simulink model "ARI_25_1_Smith_predictor"  (Simulink 7.8)
settings: Solver=ode45  StartTime=0.0  StopTime=5  RelTol=1e-3
values from neighbouring files (symbols this model uses):
  tau = tol*max(norm(y,'inf'),1.0)    [phase.m]
undefined symbols (not defined in the file or in its folder): A, B, C, D
libraries: simulink x1
settings Model: Creator=Michael Sebek  ModifiedByFormat=Michael Sebek  LastModifiedBy=Michael Sebek
settings OptimizationCC: InitFltsAndDblsToZero=on
settings DebuggingCC: SaveWithParameterizedLinksMsg=none  SignalResolutionControl=TryResolveAllWithWarning  MultiTaskDSMMsg=warning  MultiTaskCondExecSysMsg=none  FcnCallInpInsideContextMsg=Use local settings  StrictBusMsg=None
settings RTWCC: IncludeERTFirstTime=on
settings GRTTargetCC: TargetFcnLib=ansi_tfl_tmw.mat

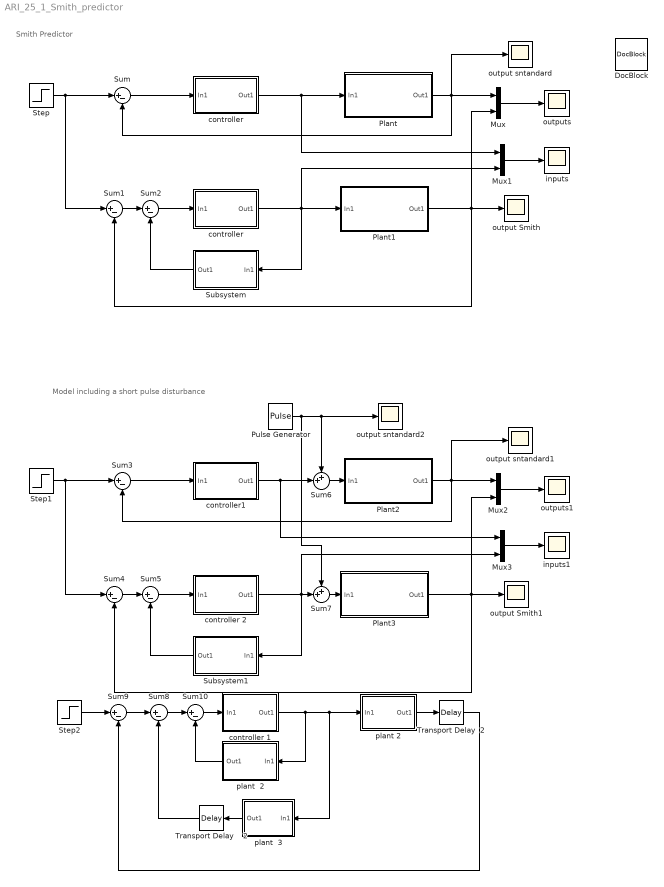
== system ARI_25_1_Smith_predictor ==
  note: Smith Predictor
  note: Model including a short pulse disturbance
  DocBlock : simulink/Model-Wide Utilities/DocBlock  DocumentType=Text
  Mux{,1..3} (4 alike) : Mux  Inputs=2
  Plant : Subsystem
      mask Display: disp('F(s)*exp(-s*tau)')
  Plant1 : Subsystem
      mask Display: disp('F(s)*exp(-s*tau)')
  Plant2 : Subsystem
      mask Display: disp('F(s)*exp(-s*tau)')
  Plant3 : Subsystem
      mask Display: disp('F(s)*exp(-s*tau)')
  Pulse Generator : DiscretePulseGenerator  PulseType=Time based  Period=100  PhaseDelay=1
  Step : Step  Time=0  SampleTime=0
  Step1 : Step  Time=0  SampleTime=0
  Step2 : Step  SampleTime=0
  Subsystem : Subsystem
      mask Display: disp('Smith')
  Subsystem1 : Subsystem
      mask Display: disp('Smith')
  Sum{,1..5,8..10} (9 alike) : Sum  Inputs=|+-
  Sum6 : Sum  Inputs=++|
  Sum7 : Sum  Inputs=++|
  Transport Delay    2 : TransportDelay
  Transport Delay  2 : TransportDelay
  controller : Subsystem  mask(PMF Block){F=C, InCon=[ ], SampTime=1, fvar=No change}
      mask prompts: F "PMF Object:"; InCon "Initial states:"; SampTime "Sample time (discrete time only):"; fvar "Force variable:"
      mask help:
      | Polynomial matrix fraction description of a linear system.
      |
      | This block represents a linear system defined by the polynomial matrix fraction of its transfer function.
      mask init:
      | Label = 'xxx';
      | [A,B,C,D,Label,var] = polymask2(F, fvar, length(InCon));
      | update;
      mask Help:
      | This block represents a linear system [<I>A,B,C,D</I>] defined by the polynomial matrix fraction (<I>PMF</I>) of its transfer function <I>T</I>.
      | <p>
      | <b>Left Matrix Fraction</b> item of the popup menu <b>Type</b> indicates the transfer function in the form of <I>left PMF</I>:
      | <p>
      | <I>T</I> = inv(<I>Q</I>) <I>P</I>.
      | <p>
      | <b>Right Matrix Fraction</b> item is used if the transfer function is given in the form of <I>right PMF</I>:
      | <p>
      | <I>T</I> = <I>P</I> inv(<I>Q</I>).
      | <p>
      |  The <b>variable</b> determines the type  of the system:
      | <p>
      | - <b>s, p</b> are used for continous time systems (Laplace transform).
      | <p>
      | - <b>z, q</b> are used for discrete time transfer functions in forward-shift operator (Z-transform).
      | <p>
      | - <b>d, z^-1</b> are used for discrete time transfer functions in backward-shift operator.
      | <p>
      | <b> Note:</b> For the variables <I>s,p,z,q</I>, the transfer function is defined as
      | <p>
      | <I>T</I> = <I>C</I> inv(<I>vI-A</I>) <I>B</I> + <I>D</I>,
      | <p>
      | where <I>v</I> is the variable of <I>P,Q</I>.
      | For the variables <I>d, z^-1</I>, the transfer function is defined as
      | <p>
      | <I>T</I> = <I>C v</I> inv(<I>I-Av</I>)  <I>B</I> + <I>D</I>.
      | <p>
      | <b>Note:</b> <b>Initial states</b> concern the observer-form realization of the system as defined by LMF2S and RMF2S functions. Their number must equal the sum of column degrees of the denominator matrix <I>Q</I> in case of right PMF and the sum of row degrees of <I>Q</I> for left PMF description.
      | <p>
      | See also POL, LMF2S, RMF2S.
      mask StyleString: edit,edit,edit,popup(No change|s   (continous time)|p   (continous time)|z      (discrete time)|q      (discrete time)|d      (discrete time)|z^-1 (discrete time))
      mask Display: disp('C(s)')
  "controller " : Subsystem  mask(PMF Block){F=C, InCon=[ ], SampTime=1, fvar=No change}
      mask prompts: F "PMF Object:"; InCon "Initial states:"; SampTime "Sample time (discrete time only):"; fvar "Force variable:"
      mask help:
      | Polynomial matrix fraction description of a linear system.
      |
      | This block represents a linear system defined by the polynomial matrix fraction of its transfer function.
      mask init:
      | Label = 'xxx';
      | [A,B,C,D,Label,var] = polymask2(F, fvar, length(InCon));
      | update;
      mask Help:
      | This block represents a linear system [<I>A,B,C,D</I>] defined by the polynomial matrix fraction (<I>PMF</I>) of its transfer function <I>T</I>.
      | <p>
      | <b>Left Matrix Fraction</b> item of the popup menu <b>Type</b> indicates the transfer function in the form of <I>left PMF</I>:
      | <p>
      | <I>T</I> = inv(<I>Q</I>) <I>P</I>.
      | <p>
      | <b>Right Matrix Fraction</b> item is used if the transfer function is given in the form of <I>right PMF</I>:
      | <p>
      | <I>T</I> = <I>P</I> inv(<I>Q</I>).
      | <p>
      |  The <b>variable</b> determines the type  of the system:
      | <p>
      | - <b>s, p</b> are used for continous time systems (Laplace transform).
      | <p>
      | - <b>z, q</b> are used for discrete time transfer functions in forward-shift operator (Z-transform).
      | <p>
      | - <b>d, z^-1</b> are used for discrete time transfer functions in backward-shift operator.
      | <p>
      | <b> Note:</b> For the variables <I>s,p,z,q</I>, the transfer function is defined as
      | <p>
      | <I>T</I> = <I>C</I> inv(<I>vI-A</I>) <I>B</I> + <I>D</I>,
      | <p>
      | where <I>v</I> is the variable of <I>P,Q</I>.
      | For the variables <I>d, z^-1</I>, the transfer function is defined as
      | <p>
      | <I>T</I> = <I>C v</I> inv(<I>I-Av</I>)  <I>B</I> + <I>D</I>.
      | <p>
      | <b>Note:</b> <b>Initial states</b> concern the observer-form realization of the system as defined by LMF2S and RMF2S functions. Their number must equal the sum of column degrees of the denominator matrix <I>Q</I> in case of right PMF and the sum of row degrees of <I>Q</I> for left PMF description.
      | <p>
      | See also POL, LMF2S, RMF2S.
      mask StyleString: edit,edit,edit,popup(No change|s   (continous time)|p   (continous time)|z      (discrete time)|q      (discrete time)|d      (discrete time)|z^-1 (discrete time))
      mask Display: disp('C(s)')
  controller 1 : Subsystem  mask(PMF Block){F=1/s, InCon=[ ], SampTime=1, fvar=No change}
      mask prompts: F "PMF Object:"; InCon "Initial states:"; SampTime "Sample time (discrete time only):"; fvar "Force variable:"
      mask help:
      | Polynomial matrix fraction description of a linear system.
      |
      | This block represents a linear system defined by the polynomial matrix fraction of its transfer function.
      mask init:
      | Label = 'xxx';
      | [A,B,C,D,Label,var] = polymask2(F, fvar, length(InCon));
      | update;
      mask Help:
      | This block represents a linear system [<I>A,B,C,D</I>] defined by the polynomial matrix fraction (<I>PMF</I>) of its transfer function <I>T</I>.
      | <p>
      | <b>Left Matrix Fraction</b> item of the popup menu <b>Type</b> indicates the transfer function in the form of <I>left PMF</I>:
      | <p>
      | <I>T</I> = inv(<I>Q</I>) <I>P</I>.
      | <p>
      | <b>Right Matrix Fraction</b> item is used if the transfer function is given in the form of <I>right PMF</I>:
      | <p>
      | <I>T</I> = <I>P</I> inv(<I>Q</I>).
      | <p>
      |  The <b>variable</b> determines the type  of the system:
      | <p>
      | - <b>s, p</b> are used for continous time systems (Laplace transform).
      | <p>
      | - <b>z, q</b> are used for discrete time transfer functions in forward-shift operator (Z-transform).
      | <p>
      | - <b>d, z^-1</b> are used for discrete time transfer functions in backward-shift operator.
      | <p>
      | <b> Note:</b> For the variables <I>s,p,z,q</I>, the transfer function is defined as
      | <p>
      | <I>T</I> = <I>C</I> inv(<I>vI-A</I>) <I>B</I> + <I>D</I>,
      | <p>
      | where <I>v</I> is the variable of <I>P,Q</I>.
      | For the variables <I>d, z^-1</I>, the transfer function is defined as
      | <p>
      | <I>T</I> = <I>C v</I> inv(<I>I-Av</I>)  <I>B</I> + <I>D</I>.
      | <p>
      | <b>Note:</b> <b>Initial states</b> concern the observer-form realization of the system as defined by LMF2S and RMF2S functions. Their number must equal the sum of column degrees of the denominator matrix <I>Q</I> in case of right PMF and the sum of row degrees of <I>Q</I> for left PMF description.
      | <p>
      | See also POL, LMF2S, RMF2S.
      mask StyleString: edit,edit,edit,popup(No change|s   (continous time)|p   (continous time)|z      (discrete time)|q      (discrete time)|d      (discrete time)|z^-1 (discrete time))
      mask Display: disp(Label);
  controller 2 : Subsystem  mask(PMF Block){F=C, InCon=[ ], SampTime=1, fvar=No change}
      mask prompts: F "PMF Object:"; InCon "Initial states:"; SampTime "Sample time (discrete time only):"; fvar "Force variable:"
      mask help:
      | Polynomial matrix fraction description of a linear system.
      |
      | This block represents a linear system defined by the polynomial matrix fraction of its transfer function.
      mask init:
      | Label = 'xxx';
      | [A,B,C,D,Label,var] = polymask2(F, fvar, length(InCon));
      | update;
      mask Help:
      | This block represents a linear system [<I>A,B,C,D</I>] defined by the polynomial matrix fraction (<I>PMF</I>) of its transfer function <I>T</I>.
      | <p>
      | <b>Left Matrix Fraction</b> item of the popup menu <b>Type</b> indicates the transfer function in the form of <I>left PMF</I>:
      | <p>
      | <I>T</I> = inv(<I>Q</I>) <I>P</I>.
      | <p>
      | <b>Right Matrix Fraction</b> item is used if the transfer function is given in the form of <I>right PMF</I>:
      | <p>
      | <I>T</I> = <I>P</I> inv(<I>Q</I>).
      | <p>
      |  The <b>variable</b> determines the type  of the system:
      | <p>
      | - <b>s, p</b> are used for continous time systems (Laplace transform).
      | <p>
      | - <b>z, q</b> are used for discrete time transfer functions in forward-shift operator (Z-transform).
      | <p>
      | - <b>d, z^-1</b> are used for discrete time transfer functions in backward-shift operator.
      | <p>
      | <b> Note:</b> For the variables <I>s,p,z,q</I>, the transfer function is defined as
      | <p>
      | <I>T</I> = <I>C</I> inv(<I>vI-A</I>) <I>B</I> + <I>D</I>,
      | <p>
      | where <I>v</I> is the variable of <I>P,Q</I>.
      | For the variables <I>d, z^-1</I>, the transfer function is defined as
      | <p>
      | <I>T</I> = <I>C v</I> inv(<I>I-Av</I>)  <I>B</I> + <I>D</I>.
      | <p>
      | <b>Note:</b> <b>Initial states</b> concern the observer-form realization of the system as defined by LMF2S and RMF2S functions. Their number must equal the sum of column degrees of the denominator matrix <I>Q</I> in case of right PMF and the sum of row degrees of <I>Q</I> for left PMF description.
      | <p>
      | See also POL, LMF2S, RMF2S.
      mask StyleString: edit,edit,edit,popup(No change|s   (continous time)|p   (continous time)|z      (discrete time)|q      (discrete time)|d      (discrete time)|z^-1 (discrete time))
      mask Display: disp('C(s)')
  controller1 : Subsystem  mask(PMF Block){F=C, InCon=[ ], SampTime=1, fvar=No change}
      mask prompts: F "PMF Object:"; InCon "Initial states:"; SampTime "Sample time (discrete time only):"; fvar "Force variable:"
      mask help:
      | Polynomial matrix fraction description of a linear system.
      |
      | This block represents a linear system defined by the polynomial matrix fraction of its transfer function.
      mask init:
      | Label = 'xxx';
      | [A,B,C,D,Label,var] = polymask2(F, fvar, length(InCon));
      | update;
      mask Help:
      | This block represents a linear system [<I>A,B,C,D</I>] defined by the polynomial matrix fraction (<I>PMF</I>) of its transfer function <I>T</I>.
      | <p>
      | <b>Left Matrix Fraction</b> item of the popup menu <b>Type</b> indicates the transfer function in the form of <I>left PMF</I>:
      | <p>
      | <I>T</I> = inv(<I>Q</I>) <I>P</I>.
      | <p>
      | <b>Right Matrix Fraction</b> item is used if the transfer function is given in the form of <I>right PMF</I>:
      | <p>
      | <I>T</I> = <I>P</I> inv(<I>Q</I>).
      | <p>
      |  The <b>variable</b> determines the type  of the system:
      | <p>
      | - <b>s, p</b> are used for continous time systems (Laplace transform).
      | <p>
      | - <b>z, q</b> are used for discrete time transfer functions in forward-shift operator (Z-transform).
      | <p>
      | - <b>d, z^-1</b> are used for discrete time transfer functions in backward-shift operator.
      | <p>
      | <b> Note:</b> For the variables <I>s,p,z,q</I>, the transfer function is defined as
      | <p>
      | <I>T</I> = <I>C</I> inv(<I>vI-A</I>) <I>B</I> + <I>D</I>,
      | <p>
      | where <I>v</I> is the variable of <I>P,Q</I>.
      | For the variables <I>d, z^-1</I>, the transfer function is defined as
      | <p>
      | <I>T</I> = <I>C v</I> inv(<I>I-Av</I>)  <I>B</I> + <I>D</I>.
      | <p>
      | <b>Note:</b> <b>Initial states</b> concern the observer-form realization of the system as defined by LMF2S and RMF2S functions. Their number must equal the sum of column degrees of the denominator matrix <I>Q</I> in case of right PMF and the sum of row degrees of <I>Q</I> for left PMF description.
      | <p>
      | See also POL, LMF2S, RMF2S.
      mask StyleString: edit,edit,edit,popup(No change|s   (continous time)|p   (continous time)|z      (discrete time)|q      (discrete time)|d      (discrete time)|z^-1 (discrete time))
      mask Display: disp('C(s)')
  inputs : Scope
      settings: SaveName=ScopeData2
  inputs1 : Scope
      settings: SaveName=ScopeData4
  output Smith : Scope
  output Smith1 : Scope
      settings: SaveName=ScopeData5
  output sntandard : Scope
      settings: SaveName=ScopeData3
  output sntandard1 : Scope
      settings: SaveName=ScopeData6
  output sntandard2 : Scope
      settings: SaveName=ScopeData8
  outputs : Scope
      settings: TimeRange=50  YMin=0  YMax=1.4e+021
  outputs1 : Scope
      settings: TimeRange=50  YMin=0  YMax=1.4e+021  SaveName=ScopeData7
  plant  2 : Subsystem  mask(PMF Block){F=rdf(1,s+1), InCon=[ ], SampTime=1, fvar=No change}
      mask prompts: F "PMF Object:"; InCon "Initial states:"; SampTime "Sample time (discrete time only):"; fvar "Force variable:"
      mask help:
      | Polynomial matrix fraction description of a linear system.
      |
      | This block represents a linear system defined by the polynomial matrix fraction of its transfer function.
      mask init:
      | Label = 'xxx';
      | [A,B,C,D,Label,var] = polymask2(F, fvar, length(InCon));
      | update;
      mask Help:
      | This block represents a linear system [<I>A,B,C,D</I>] defined by the polynomial matrix fraction (<I>PMF</I>) of its transfer function <I>T</I>.
      | <p>
      | <b>Left Matrix Fraction</b> item of the popup menu <b>Type</b> indicates the transfer function in the form of <I>left PMF</I>:
      | <p>
      | <I>T</I> = inv(<I>Q</I>) <I>P</I>.
      | <p>
      | <b>Right Matrix Fraction</b> item is used if the transfer function is given in the form of <I>right PMF</I>:
      | <p>
      | <I>T</I> = <I>P</I> inv(<I>Q</I>).
      | <p>
      |  The <b>variable</b> determines the type  of the system:
      | <p>
      | - <b>s, p</b> are used for continous time systems (Laplace transform).
      | <p>
      | - <b>z, q</b> are used for discrete time transfer functions in forward-shift operator (Z-transform).
      | <p>
      | - <b>d, z^-1</b> are used for discrete time transfer functions in backward-shift operator.
      | <p>
      | <b> Note:</b> For the variables <I>s,p,z,q</I>, the transfer function is defined as
      | <p>
      | <I>T</I> = <I>C</I> inv(<I>vI-A</I>) <I>B</I> + <I>D</I>,
      | <p>
      | where <I>v</I> is the variable of <I>P,Q</I>.
      | For the variables <I>d, z^-1</I>, the transfer function is defined as
      | <p>
      | <I>T</I> = <I>C v</I> inv(<I>I-Av</I>)  <I>B</I> + <I>D</I>.
      | <p>
      | <b>Note:</b> <b>Initial states</b> concern the observer-form realization of the system as defined by LMF2S and RMF2S functions. Their number must equal the sum of column degrees of the denominator matrix <I>Q</I> in case of right PMF and the sum of row degrees of <I>Q</I> for left PMF description.
      | <p>
      | See also POL, LMF2S, RMF2S.
      mask StyleString: edit,edit,edit,popup(No change|s   (continous time)|p   (continous time)|z      (discrete time)|q      (discrete time)|d      (discrete time)|z^-1 (discrete time))
      mask Display: disp(Label);
  plant  3 : Subsystem  mask(PMF Block){F=rdf(1,s+1), InCon=[ ], SampTime=1, fvar=No change}
      mask prompts: F "PMF Object:"; InCon "Initial states:"; SampTime "Sample time (discrete time only):"; fvar "Force variable:"
      mask help:
      | Polynomial matrix fraction description of a linear system.
      |
      | This block represents a linear system defined by the polynomial matrix fraction of its transfer function.
      mask init:
      | Label = 'xxx';
      | [A,B,C,D,Label,var] = polymask2(F, fvar, length(InCon));
      | update;
      mask Help:
      | This block represents a linear system [<I>A,B,C,D</I>] defined by the polynomial matrix fraction (<I>PMF</I>) of its transfer function <I>T</I>.
      | <p>
      | <b>Left Matrix Fraction</b> item of the popup menu <b>Type</b> indicates the transfer function in the form of <I>left PMF</I>:
      | <p>
      | <I>T</I> = inv(<I>Q</I>) <I>P</I>.
      | <p>
      | <b>Right Matrix Fraction</b> item is used if the transfer function is given in the form of <I>right PMF</I>:
      | <p>
      | <I>T</I> = <I>P</I> inv(<I>Q</I>).
      | <p>
      |  The <b>variable</b> determines the type  of the system:
      | <p>
      | - <b>s, p</b> are used for continous time systems (Laplace transform).
      | <p>
      | - <b>z, q</b> are used for discrete time transfer functions in forward-shift operator (Z-transform).
      | <p>
      | - <b>d, z^-1</b> are used for discrete time transfer functions in backward-shift operator.
      | <p>
      | <b> Note:</b> For the variables <I>s,p,z,q</I>, the transfer function is defined as
      | <p>
      | <I>T</I> = <I>C</I> inv(<I>vI-A</I>) <I>B</I> + <I>D</I>,
      | <p>
      | where <I>v</I> is the variable of <I>P,Q</I>.
      | For the variables <I>d, z^-1</I>, the transfer function is defined as
      | <p>
      | <I>T</I> = <I>C v</I> inv(<I>I-Av</I>)  <I>B</I> + <I>D</I>.
      | <p>
      | <b>Note:</b> <b>Initial states</b> concern the observer-form realization of the system as defined by LMF2S and RMF2S functions. Their number must equal the sum of column degrees of the denominator matrix <I>Q</I> in case of right PMF and the sum of row degrees of <I>Q</I> for left PMF description.
      | <p>
      | See also POL, LMF2S, RMF2S.
      mask StyleString: edit,edit,edit,popup(No change|s   (continous time)|p   (continous time)|z      (discrete time)|q      (discrete time)|d      (discrete time)|z^-1 (discrete time))
      mask Display: disp(Label);
  plant 2 : Subsystem  mask(PMF Block){F=rdf(1,s+1), InCon=[ ], SampTime=1, fvar=No change}
      mask prompts: F "PMF Object:"; InCon "Initial states:"; SampTime "Sample time (discrete time only):"; fvar "Force variable:"
      mask help:
      | Polynomial matrix fraction description of a linear system.
      |
      | This block represents a linear system defined by the polynomial matrix fraction of its transfer function.
      mask init:
      | Label = 'xxx';
      | [A,B,C,D,Label,var] = polymask2(F, fvar, length(InCon));
      | update;
      mask Help:
      | This block represents a linear system [<I>A,B,C,D</I>] defined by the polynomial matrix fraction (<I>PMF</I>) of its transfer function <I>T</I>.
      | <p>
      | <b>Left Matrix Fraction</b> item of the popup menu <b>Type</b> indicates the transfer function in the form of <I>left PMF</I>:
      | <p>
      | <I>T</I> = inv(<I>Q</I>) <I>P</I>.
      | <p>
      | <b>Right Matrix Fraction</b> item is used if the transfer function is given in the form of <I>right PMF</I>:
      | <p>
      | <I>T</I> = <I>P</I> inv(<I>Q</I>).
      | <p>
      |  The <b>variable</b> determines the type  of the system:
      | <p>
      | - <b>s, p</b> are used for continous time systems (Laplace transform).
      | <p>
      | - <b>z, q</b> are used for discrete time transfer functions in forward-shift operator (Z-transform).
      | <p>
      | - <b>d, z^-1</b> are used for discrete time transfer functions in backward-shift operator.
      | <p>
      | <b> Note:</b> For the variables <I>s,p,z,q</I>, the transfer function is defined as
      | <p>
      | <I>T</I> = <I>C</I> inv(<I>vI-A</I>) <I>B</I> + <I>D</I>,
      | <p>
      | where <I>v</I> is the variable of <I>P,Q</I>.
      | For the variables <I>d, z^-1</I>, the transfer function is defined as
      | <p>
      | <I>T</I> = <I>C v</I> inv(<I>I-Av</I>)  <I>B</I> + <I>D</I>.
      | <p>
      | <b>Note:</b> <b>Initial states</b> concern the observer-form realization of the system as defined by LMF2S and RMF2S functions. Their number must equal the sum of column degrees of the denominator matrix <I>Q</I> in case of right PMF and the sum of row degrees of <I>Q</I> for left PMF description.
      | <p>
      | See also POL, LMF2S, RMF2S.
      mask StyleString: edit,edit,edit,popup(No change|s   (continous time)|p   (continous time)|z      (discrete time)|q      (discrete time)|d      (discrete time)|z^-1 (discrete time))
      mask Display: droots([], [-1], 1)
  wires:
  Mux/1 -> outputs/1
  Plant/1(Out1) -> Mux/1, Sum/2, output sntandard/1
  controller/1(Out1) -> Plant/1(In1), Mux1/1
  Sum/1 -> controller/1(In1)
  Step/1 -> Sum/1, Sum1/1
  "controller "/1(Out1) -> Plant1/1(In1), Subsystem/1(In1), Mux1/2
  Sum2/1 -> "controller "/1(In1)
  Subsystem/1(Out1) -> Sum2/2
  plant 2/1(Out1) -> Transport Delay  2/1
  controller 1/1(Out1) -> plant  2/1(In1), plant 2/1(In1), plant  3/1(In1)
  Sum10/1 -> controller 1/1(In1)
  plant  2/1(Out1) -> Sum10/2
  Transport Delay  2/1 -> Sum9/2
  Step2/1 -> Sum9/1
  plant  3/1(Out1) -> Transport Delay    2/1
  Sum8/1 -> Sum10/1
  Sum9/1 -> Sum8/1
  Transport Delay    2/1 -> Sum8/2
  Plant1/1(Out1) -> Sum1/2, output Smith/1, Mux/2
  Mux1/1 -> inputs/1
  Sum1/1 -> Sum2/1
  Mux2/1 -> outputs1/1
  Plant2/1(Out1) -> output sntandard1/1, Sum3/2, Mux2/1
  Sum3/1 -> controller1/1(In1)
  Step1/1 -> Sum4/1, Sum3/1
  Sum5/1 -> controller 2/1(In1)
  Subsystem1/1(Out1) -> Sum5/2
  Plant3/1(Out1) -> Mux2/2, output Smith1/1, Sum4/2
  Mux3/1 -> inputs1/1
  Sum4/1 -> Sum5/1
  controller1/1(Out1) -> Sum6/2, Mux3/1
  Sum6/1 -> Plant2/1(In1)
  Pulse Generator/1 -> Sum6/1, output sntandard2/1, Sum7/1
  controller 2/1(Out1) -> Mux3/2, Subsystem1/1(In1), Sum7/2
  Sum7/1 -> Plant3/1(In1)

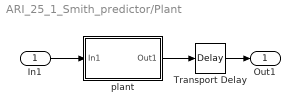
== system ARI_25_1_Smith_predictor/Plant ==
  In1 : Inport
  Transport Delay : TransportDelay  DelayTime=tau
  plant : Subsystem  mask(PMF Block){F=F, InCon=[ ], SampTime=1, fvar=No change}
      mask prompts: F "PMF Object:"; InCon "Initial states:"; SampTime "Sample time (discrete time only):"; fvar "Force variable:"
      mask help:
      | Polynomial matrix fraction description of a linear system.
      |
      | This block represents a linear system defined by the polynomial matrix fraction of its transfer function.
      mask init:
      | Label = 'xxx';
      | [A,B,C,D,Label,var] = polymask2(F, fvar, length(InCon));
      | update;
      mask Help:
      | This block represents a linear system [<I>A,B,C,D</I>] defined by the polynomial matrix fraction (<I>PMF</I>) of its transfer function <I>T</I>.
      | <p>
      | <b>Left Matrix Fraction</b> item of the popup menu <b>Type</b> indicates the transfer function in the form of <I>left PMF</I>:
      | <p>
      | <I>T</I> = inv(<I>Q</I>) <I>P</I>.
      | <p>
      | <b>Right Matrix Fraction</b> item is used if the transfer function is given in the form of <I>right PMF</I>:
      | <p>
      | <I>T</I> = <I>P</I> inv(<I>Q</I>).
      | <p>
      |  The <b>variable</b> determines the type  of the system:
      | <p>
      | - <b>s, p</b> are used for continous time systems (Laplace transform).
      | <p>
      | - <b>z, q</b> are used for discrete time transfer functions in forward-shift operator (Z-transform).
      | <p>
      | - <b>d, z^-1</b> are used for discrete time transfer functions in backward-shift operator.
      | <p>
      | <b> Note:</b> For the variables <I>s,p,z,q</I>, the transfer function is defined as
      | <p>
      | <I>T</I> = <I>C</I> inv(<I>vI-A</I>) <I>B</I> + <I>D</I>,
      | <p>
      | where <I>v</I> is the variable of <I>P,Q</I>.
      | For the variables <I>d, z^-1</I>, the transfer function is defined as
      | <p>
      | <I>T</I> = <I>C v</I> inv(<I>I-Av</I>)  <I>B</I> + <I>D</I>.
      | <p>
      | <b>Note:</b> <b>Initial states</b> concern the observer-form realization of the system as defined by LMF2S and RMF2S functions. Their number must equal the sum of column degrees of the denominator matrix <I>Q</I> in case of right PMF and the sum of row degrees of <I>Q</I> for left PMF description.
      | <p>
      | See also POL, LMF2S, RMF2S.
      mask StyleString: edit,edit,edit,popup(No change|s   (continous time)|p   (continous time)|z      (discrete time)|q      (discrete time)|d      (discrete time)|z^-1 (discrete time))
      mask Display: disp('F(s)')
  Out1 : Outport
  wires:
  plant/1(Out1) -> Transport Delay/1
  In1/1 -> plant/1(In1)
  Transport Delay/1 -> Out1/1

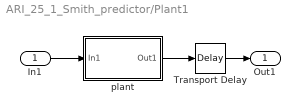
== system ARI_25_1_Smith_predictor/Plant1 ==
  In1 : Inport
  Transport Delay : TransportDelay  DelayTime=tau
  plant : Subsystem  mask(PMF Block){F=F, InCon=[ ], SampTime=1, fvar=No change}
      mask prompts: F "PMF Object:"; InCon "Initial states:"; SampTime "Sample time (discrete time only):"; fvar "Force variable:"
      mask help:
      | Polynomial matrix fraction description of a linear system.
      |
      | This block represents a linear system defined by the polynomial matrix fraction of its transfer function.
      mask init:
      | Label = 'xxx';
      | [A,B,C,D,Label,var] = polymask2(F, fvar, length(InCon));
      | update;
      mask Help:
      | This block represents a linear system [<I>A,B,C,D</I>] defined by the polynomial matrix fraction (<I>PMF</I>) of its transfer function <I>T</I>.
      | <p>
      | <b>Left Matrix Fraction</b> item of the popup menu <b>Type</b> indicates the transfer function in the form of <I>left PMF</I>:
      | <p>
      | <I>T</I> = inv(<I>Q</I>) <I>P</I>.
      | <p>
      | <b>Right Matrix Fraction</b> item is used if the transfer function is given in the form of <I>right PMF</I>:
      | <p>
      | <I>T</I> = <I>P</I> inv(<I>Q</I>).
      | <p>
      |  The <b>variable</b> determines the type  of the system:
      | <p>
      | - <b>s, p</b> are used for continous time systems (Laplace transform).
      | <p>
      | - <b>z, q</b> are used for discrete time transfer functions in forward-shift operator (Z-transform).
      | <p>
      | - <b>d, z^-1</b> are used for discrete time transfer functions in backward-shift operator.
      | <p>
      | <b> Note:</b> For the variables <I>s,p,z,q</I>, the transfer function is defined as
      | <p>
      | <I>T</I> = <I>C</I> inv(<I>vI-A</I>) <I>B</I> + <I>D</I>,
      | <p>
      | where <I>v</I> is the variable of <I>P,Q</I>.
      | For the variables <I>d, z^-1</I>, the transfer function is defined as
      | <p>
      | <I>T</I> = <I>C v</I> inv(<I>I-Av</I>)  <I>B</I> + <I>D</I>.
      | <p>
      | <b>Note:</b> <b>Initial states</b> concern the observer-form realization of the system as defined by LMF2S and RMF2S functions. Their number must equal the sum of column degrees of the denominator matrix <I>Q</I> in case of right PMF and the sum of row degrees of <I>Q</I> for left PMF description.
      | <p>
      | See also POL, LMF2S, RMF2S.
      mask StyleString: edit,edit,edit,popup(No change|s   (continous time)|p   (continous time)|z      (discrete time)|q      (discrete time)|d      (discrete time)|z^-1 (discrete time))
      mask Display: disp('b/a')
  Out1 : Outport
  wires:
  Transport Delay/1 -> Out1/1
  In1/1 -> plant/1(In1)
  plant/1(Out1) -> Transport Delay/1

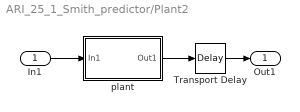
== system ARI_25_1_Smith_predictor/Plant2 ==
  In1 : Inport
  Transport Delay : TransportDelay  DelayTime=tau
  plant : Subsystem  mask(PMF Block){F=F, InCon=[ ], SampTime=1, fvar=No change}
      mask prompts: F "PMF Object:"; InCon "Initial states:"; SampTime "Sample time (discrete time only):"; fvar "Force variable:"
      mask help:
      | Polynomial matrix fraction description of a linear system.
      |
      | This block represents a linear system defined by the polynomial matrix fraction of its transfer function.
      mask init:
      | Label = 'xxx';
      | [A,B,C,D,Label,var] = polymask2(F, fvar, length(InCon));
      | update;
      mask Help:
      | This block represents a linear system [<I>A,B,C,D</I>] defined by the polynomial matrix fraction (<I>PMF</I>) of its transfer function <I>T</I>.
      | <p>
      | <b>Left Matrix Fraction</b> item of the popup menu <b>Type</b> indicates the transfer function in the form of <I>left PMF</I>:
      | <p>
      | <I>T</I> = inv(<I>Q</I>) <I>P</I>.
      | <p>
      | <b>Right Matrix Fraction</b> item is used if the transfer function is given in the form of <I>right PMF</I>:
      | <p>
      | <I>T</I> = <I>P</I> inv(<I>Q</I>).
      | <p>
      |  The <b>variable</b> determines the type  of the system:
      | <p>
      | - <b>s, p</b> are used for continous time systems (Laplace transform).
      | <p>
      | - <b>z, q</b> are used for discrete time transfer functions in forward-shift operator (Z-transform).
      | <p>
      | - <b>d, z^-1</b> are used for discrete time transfer functions in backward-shift operator.
      | <p>
      | <b> Note:</b> For the variables <I>s,p,z,q</I>, the transfer function is defined as
      | <p>
      | <I>T</I> = <I>C</I> inv(<I>vI-A</I>) <I>B</I> + <I>D</I>,
      | <p>
      | where <I>v</I> is the variable of <I>P,Q</I>.
      | For the variables <I>d, z^-1</I>, the transfer function is defined as
      | <p>
      | <I>T</I> = <I>C v</I> inv(<I>I-Av</I>)  <I>B</I> + <I>D</I>.
      | <p>
      | <b>Note:</b> <b>Initial states</b> concern the observer-form realization of the system as defined by LMF2S and RMF2S functions. Their number must equal the sum of column degrees of the denominator matrix <I>Q</I> in case of right PMF and the sum of row degrees of <I>Q</I> for left PMF description.
      | <p>
      | See also POL, LMF2S, RMF2S.
      mask StyleString: edit,edit,edit,popup(No change|s   (continous time)|p   (continous time)|z      (discrete time)|q      (discrete time)|d      (discrete time)|z^-1 (discrete time))
      mask Display: disp('F(s)')
  Out1 : Outport
  wires:
  Transport Delay/1 -> Out1/1
  In1/1 -> plant/1(In1)
  plant/1(Out1) -> Transport Delay/1

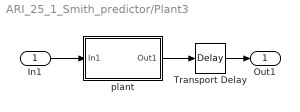
== system ARI_25_1_Smith_predictor/Plant3 ==
  In1 : Inport
  Transport Delay : TransportDelay  DelayTime=tau
  plant : Subsystem  mask(PMF Block){F=F, InCon=[ ], SampTime=1, fvar=No change}
      mask prompts: F "PMF Object:"; InCon "Initial states:"; SampTime "Sample time (discrete time only):"; fvar "Force variable:"
      mask help:
      | Polynomial matrix fraction description of a linear system.
      |
      | This block represents a linear system defined by the polynomial matrix fraction of its transfer function.
      mask init:
      | Label = 'xxx';
      | [A,B,C,D,Label,var] = polymask2(F, fvar, length(InCon));
      | update;
      mask Help:
      | This block represents a linear system [<I>A,B,C,D</I>] defined by the polynomial matrix fraction (<I>PMF</I>) of its transfer function <I>T</I>.
      | <p>
      | <b>Left Matrix Fraction</b> item of the popup menu <b>Type</b> indicates the transfer function in the form of <I>left PMF</I>:
      | <p>
      | <I>T</I> = inv(<I>Q</I>) <I>P</I>.
      | <p>
      | <b>Right Matrix Fraction</b> item is used if the transfer function is given in the form of <I>right PMF</I>:
      | <p>
      | <I>T</I> = <I>P</I> inv(<I>Q</I>).
      | <p>
      |  The <b>variable</b> determines the type  of the system:
      | <p>
      | - <b>s, p</b> are used for continous time systems (Laplace transform).
      | <p>
      | - <b>z, q</b> are used for discrete time transfer functions in forward-shift operator (Z-transform).
      | <p>
      | - <b>d, z^-1</b> are used for discrete time transfer functions in backward-shift operator.
      | <p>
      | <b> Note:</b> For the variables <I>s,p,z,q</I>, the transfer function is defined as
      | <p>
      | <I>T</I> = <I>C</I> inv(<I>vI-A</I>) <I>B</I> + <I>D</I>,
      | <p>
      | where <I>v</I> is the variable of <I>P,Q</I>.
      | For the variables <I>d, z^-1</I>, the transfer function is defined as
      | <p>
      | <I>T</I> = <I>C v</I> inv(<I>I-Av</I>)  <I>B</I> + <I>D</I>.
      | <p>
      | <b>Note:</b> <b>Initial states</b> concern the observer-form realization of the system as defined by LMF2S and RMF2S functions. Their number must equal the sum of column degrees of the denominator matrix <I>Q</I> in case of right PMF and the sum of row degrees of <I>Q</I> for left PMF description.
      | <p>
      | See also POL, LMF2S, RMF2S.
      mask StyleString: edit,edit,edit,popup(No change|s   (continous time)|p   (continous time)|z      (discrete time)|q      (discrete time)|d      (discrete time)|z^-1 (discrete time))
      mask Display: disp('b/a')
  Out1 : Outport
  wires:
  plant/1(Out1) -> Transport Delay/1
  In1/1 -> plant/1(In1)
  Transport Delay/1 -> Out1/1

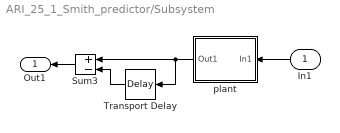
== system ARI_25_1_Smith_predictor/Subsystem ==
  In1 : Inport
  Sum3 : Sum  Inputs=+-
  "Transport Delay    " : TransportDelay  DelayTime=tau
  "plant  " : Subsystem  mask(PMF Block){F=F, InCon=[ ], SampTime=1, fvar=No change}
      mask prompts: F "PMF Object:"; InCon "Initial states:"; SampTime "Sample time (discrete time only):"; fvar "Force variable:"
      mask help:
      | Polynomial matrix fraction description of a linear system.
      |
      | This block represents a linear system defined by the polynomial matrix fraction of its transfer function.
      mask init:
      | Label = 'xxx';
      | [A,B,C,D,Label,var] = polymask2(F, fvar, length(InCon));
      | update;
      mask Help:
      | This block represents a linear system [<I>A,B,C,D</I>] defined by the polynomial matrix fraction (<I>PMF</I>) of its transfer function <I>T</I>.
      | <p>
      | <b>Left Matrix Fraction</b> item of the popup menu <b>Type</b> indicates the transfer function in the form of <I>left PMF</I>:
      | <p>
      | <I>T</I> = inv(<I>Q</I>) <I>P</I>.
      | <p>
      | <b>Right Matrix Fraction</b> item is used if the transfer function is given in the form of <I>right PMF</I>:
      | <p>
      | <I>T</I> = <I>P</I> inv(<I>Q</I>).
      | <p>
      |  The <b>variable</b> determines the type  of the system:
      | <p>
      | - <b>s, p</b> are used for continous time systems (Laplace transform).
      | <p>
      | - <b>z, q</b> are used for discrete time transfer functions in forward-shift operator (Z-transform).
      | <p>
      | - <b>d, z^-1</b> are used for discrete time transfer functions in backward-shift operator.
      | <p>
      | <b> Note:</b> For the variables <I>s,p,z,q</I>, the transfer function is defined as
      | <p>
      | <I>T</I> = <I>C</I> inv(<I>vI-A</I>) <I>B</I> + <I>D</I>,
      | <p>
      | where <I>v</I> is the variable of <I>P,Q</I>.
      | For the variables <I>d, z^-1</I>, the transfer function is defined as
      | <p>
      | <I>T</I> = <I>C v</I> inv(<I>I-Av</I>)  <I>B</I> + <I>D</I>.
      | <p>
      | <b>Note:</b> <b>Initial states</b> concern the observer-form realization of the system as defined by LMF2S and RMF2S functions. Their number must equal the sum of column degrees of the denominator matrix <I>Q</I> in case of right PMF and the sum of row degrees of <I>Q</I> for left PMF description.
      | <p>
      | See also POL, LMF2S, RMF2S.
      mask StyleString: edit,edit,edit,popup(No change|s   (continous time)|p   (continous time)|z      (discrete time)|q      (discrete time)|d      (discrete time)|z^-1 (discrete time))
      mask Display: disp('F(s)')
  Out1 : Outport
  wires:
  "plant  "/1(Out1) -> "Transport Delay    "/1, Sum3/1
  "Transport Delay    "/1 -> Sum3/2
  In1/1 -> "plant  "/1(In1)
  Sum3/1 -> Out1/1

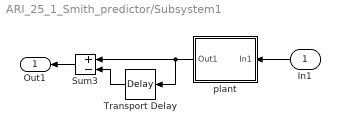
== system ARI_25_1_Smith_predictor/Subsystem1 ==
  In1 : Inport
  Sum3 : Sum  Inputs=+-
  "Transport Delay    " : TransportDelay  DelayTime=tau
  "plant  " : Subsystem  mask(PMF Block){F=F, InCon=[ ], SampTime=1, fvar=No change}
      mask prompts: F "PMF Object:"; InCon "Initial states:"; SampTime "Sample time (discrete time only):"; fvar "Force variable:"
      mask help:
      | Polynomial matrix fraction description of a linear system.
      |
      | This block represents a linear system defined by the polynomial matrix fraction of its transfer function.
      mask init:
      | Label = 'xxx';
      | [A,B,C,D,Label,var] = polymask2(F, fvar, length(InCon));
      | update;
      mask Help:
      | This block represents a linear system [<I>A,B,C,D</I>] defined by the polynomial matrix fraction (<I>PMF</I>) of its transfer function <I>T</I>.
      | <p>
      | <b>Left Matrix Fraction</b> item of the popup menu <b>Type</b> indicates the transfer function in the form of <I>left PMF</I>:
      | <p>
      | <I>T</I> = inv(<I>Q</I>) <I>P</I>.
      | <p>
      | <b>Right Matrix Fraction</b> item is used if the transfer function is given in the form of <I>right PMF</I>:
      | <p>
      | <I>T</I> = <I>P</I> inv(<I>Q</I>).
      | <p>
      |  The <b>variable</b> determines the type  of the system:
      | <p>
      | - <b>s, p</b> are used for continous time systems (Laplace transform).
      | <p>
      | - <b>z, q</b> are used for discrete time transfer functions in forward-shift operator (Z-transform).
      | <p>
      | - <b>d, z^-1</b> are used for discrete time transfer functions in backward-shift operator.
      | <p>
      | <b> Note:</b> For the variables <I>s,p,z,q</I>, the transfer function is defined as
      | <p>
      | <I>T</I> = <I>C</I> inv(<I>vI-A</I>) <I>B</I> + <I>D</I>,
      | <p>
      | where <I>v</I> is the variable of <I>P,Q</I>.
      | For the variables <I>d, z^-1</I>, the transfer function is defined as
      | <p>
      | <I>T</I> = <I>C v</I> inv(<I>I-Av</I>)  <I>B</I> + <I>D</I>.
      | <p>
      | <b>Note:</b> <b>Initial states</b> concern the observer-form realization of the system as defined by LMF2S and RMF2S functions. Their number must equal the sum of column degrees of the denominator matrix <I>Q</I> in case of right PMF and the sum of row degrees of <I>Q</I> for left PMF description.
      | <p>
      | See also POL, LMF2S, RMF2S.
      mask StyleString: edit,edit,edit,popup(No change|s   (continous time)|p   (continous time)|z      (discrete time)|q      (discrete time)|d      (discrete time)|z^-1 (discrete time))
      mask Display: disp('F(s)')
  Out1 : Outport
  wires:
  Sum3/1 -> Out1/1
  In1/1 -> "plant  "/1(In1)
  "Transport Delay    "/1 -> Sum3/2
  "plant  "/1(Out1) -> Sum3/1, "Transport Delay    "/1

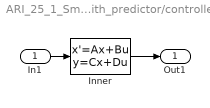
== system ARI_25_1_Smith_predictor/controller ==
  In1 : Inport
  Inner : StateSpace  A=A  B=B  C=C  D=D  X0=InCon
  Out1 : Outport
  wires:
  In1/1 -> Inner/1
  Inner/1 -> Out1/1

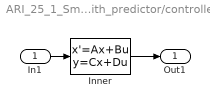
== system ARI_25_1_Smith_predictor/controller  ==
  In1 : Inport
  Inner : StateSpace  A=A  B=B  C=C  D=D  X0=InCon
  Out1 : Outport
  wires:
  Inner/1 -> Out1/1
  In1/1 -> Inner/1

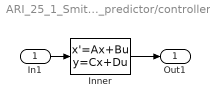
== system ARI_25_1_Smith_predictor/controller 1 ==
  In1 : Inport
  Inner : StateSpace  A=A  B=B  C=C  D=D  X0=InCon
  Out1 : Outport
  wires:
  Inner/1 -> Out1/1
  In1/1 -> Inner/1

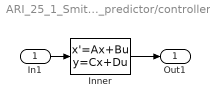
== system ARI_25_1_Smith_predictor/controller 2 ==
  In1 : Inport
  Inner : StateSpace  A=A  B=B  C=C  D=D  X0=InCon
  Out1 : Outport
  wires:
  In1/1 -> Inner/1
  Inner/1 -> Out1/1

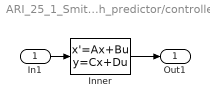
== system ARI_25_1_Smith_predictor/controller1 ==
  In1 : Inport
  Inner : StateSpace  A=A  B=B  C=C  D=D  X0=InCon
  Out1 : Outport
  wires:
  Inner/1 -> Out1/1
  In1/1 -> Inner/1

== system ARI_25_1_Smith_predictor/plant  2 ==
  In1 : Inport
  Inner : StateSpace  A=A  B=B  C=C  D=D  X0=InCon
  Out1 : Outport
  wires:
  Inner/1 -> Out1/1
  In1/1 -> Inner/1

== system ARI_25_1_Smith_predictor/plant  3 ==
  In1 : Inport
  Inner : StateSpace  A=A  B=B  C=C  D=D  X0=InCon
  Out1 : Outport
  wires:
  In1/1 -> Inner/1
  Inner/1 -> Out1/1

== system ARI_25_1_Smith_predictor/plant 2 ==
  In1 : Inport
  Inner : StateSpace  A=A  B=B  C=C  D=D  X0=InCon
  Out1 : Outport
  wires:
  In1/1 -> Inner/1
  Inner/1 -> Out1/1

== system ARI_25_1_Smith_predictor/Plant/plant ==
  In1 : Inport
  Inner : StateSpace  A=A  B=B  C=C  D=D  X0=InCon
  Out1 : Outport
  wires:
  Inner/1 -> Out1/1
  In1/1 -> Inner/1

== system ARI_25_1_Smith_predictor/Plant1/plant ==
  In1 : Inport
  Inner : StateSpace  A=A  B=B  C=C  D=D  X0=InCon
  Out1 : Outport
  wires:
  In1/1 -> Inner/1
  Inner/1 -> Out1/1

== system ARI_25_1_Smith_predictor/Plant2/plant ==
  In1 : Inport
  Inner : StateSpace  A=A  B=B  C=C  D=D  X0=InCon
  Out1 : Outport
  wires:
  In1/1 -> Inner/1
  Inner/1 -> Out1/1

== system ARI_25_1_Smith_predictor/Plant3/plant ==
  In1 : Inport
  Inner : StateSpace  A=A  B=B  C=C  D=D  X0=InCon
  Out1 : Outport
  wires:
  Inner/1 -> Out1/1
  In1/1 -> Inner/1

== system ARI_25_1_Smith_predictor/Subsystem/plant   ==
  In1 : Inport
  Inner : StateSpace  A=A  B=B  C=C  D=D  X0=InCon
  Out1 : Outport
  wires:
  Inner/1 -> Out1/1
  In1/1 -> Inner/1

== system ARI_25_1_Smith_predictor/Subsystem1/plant   ==
  In1 : Inport
  Inner : StateSpace  A=A  B=B  C=C  D=D  X0=InCon
  Out1 : Outport
  wires:
  In1/1 -> Inner/1
  Inner/1 -> Out1/1
